simulink model "lab5_sim"  (R2020a)
settings: Solver=VariableStepAuto  StartTime=0.0  StopTime=0.2  RelTol=1e-3
settings Model: Creator=milesalderman  LastModifiedBy=milesalderman
settings DebuggingCC: UnconnectedInputMsg=none  UnconnectedOutputMsg=none  UnconnectedLineMsg=none  SFMachineParentedDataDiag=error

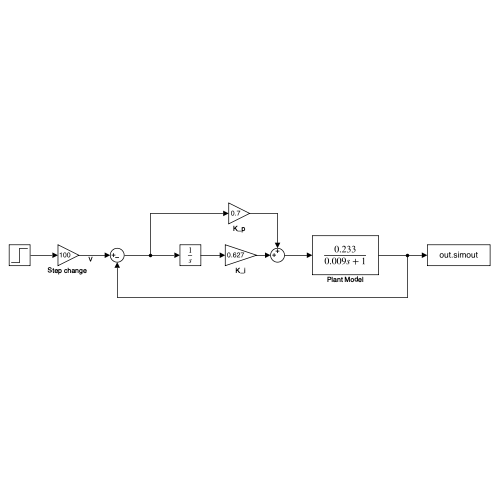
[thumbnail: Simulink's stored preview of the top-level diagram]
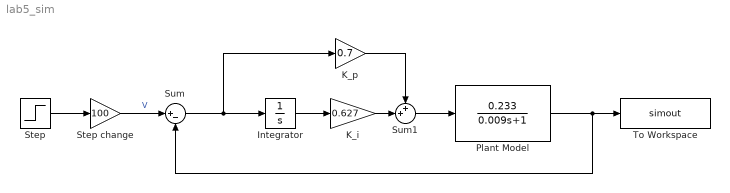
== system lab5_sim ==
  Integrator : Integrator
  K_i : Gain  Gain=0.627
  K_p : Gain  Gain=0.7
  Plant Model : TransferFcn  Numerator=[0.233]  Denominator=[0.009 1]
  Step : Step  Time=0.01  SampleTime=0
  "Step change " : Gain  Gain=100
  Sum : Sum  Inputs=|+-
  Sum1 : Sum  Inputs=++|
  To Workspace : ToWorkspace  VariableName=simout  SampleTime=-1
  wires:
  "Step change "/1 -> Sum/1  "V"
  Integrator/1 -> K_i/1
  K_p/1 -> Sum1/1
  Sum1/1 -> Plant Model/1
  Sum/1 -> Integrator/1, K_p/1
  K_i/1 -> Sum1/2
  Plant Model/1 -> To Workspace/1, Sum/2
  Step/1 -> "Step change "/1
